simulink model "ac_mode_logic"  (R2020b)
settings: Solver=VariableStepAuto  StartTime=0.0  StopTime=10.0  RelTol=1e-3
settings Model: DataDictionary=airsys_data_dict.sldd  EnableAccessToBaseWorkspace=off  Creator=Litao  LastModifiedBy=Litao

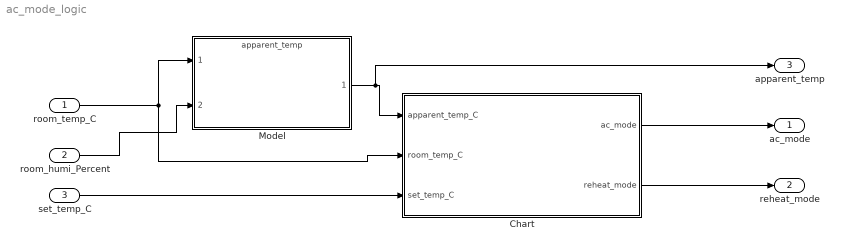
== system ac_mode_logic ==
  room_temp_C : Inport  OutDataTypeStr=double
  room_humi_Percent : Inport  Port=2  OutDataTypeStr=double
  set_temp_C : Inport  Port=3  OutDataTypeStr=double
  Chart : Stateflow chart  TreatAsAtomicUnit=on
  Model : ModelReference  ModelNameDialog=apparent_temp.slx  SimulationMode=Normal  ModelReferenceVersion=1.3
  ac_mode : Outport
  reheat_mode : Outport  Port=2
  apparent_temp : Outport  Port=3
  wires:
  room_temp_C/1 -> Model/1, Chart/2(room_temp_C)
  room_humi_Percent/1 -> Model/2
  set_temp_C/1 -> Chart/3(set_temp_C)
  Model/1 -> apparent_temp/1, Chart/1(apparent_temp_C)
  Chart/1(ac_mode) -> ac_mode/1
  Chart/2(reheat_mode) -> reheat_mode/1

== stateflow chart ac_mode_logic/Chart ==
  state Cold
    en: ac_mode = ac_mode_enum.cold
    state reheat_off
      en:reheat_mode=0;
    state reheat_on
      en:reheat_mode = 1;
      ex:reheat_mode = 0;
    (default) -> reheat_off
    reheat_on -> reheat_off : [room_temp_C-1.5>set_temp_C]
    reheat_off -> reheat_on : [room_temp_C-0.5<set_temp_C]
  state Stop
    en: ac_mode = ac_mode_enum.stop
  state Init
    en: ac_mode = ac_mode_enum.stop
  state Hot
    en: ac_mode = ac_mode_enum.hot
  Stop -> Cold [order 1] : [apparent_temp_C - set_temp_C>1.5]
  Cold -> Stop : [set_temp_C - apparent_temp_C>1]
  (default) -> Init
  Init -> Stop : [after(15,sec)]
  Hot -> Stop : [apparent_temp_C - set_temp_C>1]
  Stop -> Hot [order 2] : [set_temp_C - apparent_temp_C>1.5]
  data: apparent_temp_C input; room_temp_C input; set_temp_C input; ac_mode output; reheat_mode output
